simulink model "saturn_thermal5"  (R2021a)
settings: Solver=ode23t  StartTime=0.0  StopTime=t_simul  MaxStep=3600  MinStep=1  RelTol=0.1
values from neighbouring files (symbols this model uses):
  Ab = L*l    [Data_ini_thermal_analysis4.m]    (also in Data_ini_thermal_analysis5.m)
  Ant_Heater_MaxPower = 250    [Data_ini_thermal_analysis5.m]
  As = l*l    [Data_ini_thermal_analysis4.m]    (also in Data_ini_thermal_analysis5.m)
  D_st = 1224526    [Data_ini_thermal_analysis4.m]    (also in Data_ini_thermal_analysis5.m)
  ecc_sc = 0    [Data_ini_thermal_analysis4.m]    (also in Data_ini_thermal_analysis5.m)
  ecc_t = 0.0293    [Data_ini_thermal_analysis4.m]    (also in Data_ini_thermal_analysis5.m)
  Gr_al = sigma*epsilon_al*F_ds    (= 4.3092e-08)    [Data_ini_thermal_analysis4.m]    (also in Data_ini_thermal_analysis5.m)
  incl_ax_s = deg2rad(26.73)    [Data_ini_thermal_analysis4.m]    (also in Data_ini_thermal_analysis5.m)
  incl_sc = deg2rad(90+45)    [Data_ini_thermal_analysis4.m]    (also in Data_ini_thermal_analysis5.m)
  incl_t = deg2rad(0.3485)    [Data_ini_thermal_analysis4.m]    (also in Data_ini_thermal_analysis5.m)
  mean_motion_sc = 2*pi/period_sc    [Data_ini_thermal_analysis4.m]    (also in Data_ini_thermal_analysis5.m)
  mean_motion_t = (2*pi)/period_t    (= 4.56068561416e-06)    [Data_ini_thermal_analysis4.m]    (also in Data_ini_thermal_analysis5.m)
  mean_r_s = 1.427*10^9    (= 1427000000)    [Data_ini_thermal_analysis4.m]    (also in Data_ini_thermal_analysis5.m)
  mu_s = 37931187    [Data_ini_thermal_analysis4.m]    (also in Data_ini_thermal_analysis5.m)
  mu_t = 8971.15    [Data_ini_thermal_analysis4.m]    (also in Data_ini_thermal_analysis5.m)
  period_s = 29.45*365*24*3600    (= 928735200)    [Data_ini_thermal_analysis4.m]    (also in Data_ini_thermal_analysis5.m)
  period_t = 15.945421*24*3600    (= 1377684.3744)    [Data_ini_thermal_analysis4.m]    (also in Data_ini_thermal_analysis5.m)
  R_s = diam_s/2    (= 60268)    [Data_ini_thermal_analysis4.m]    (also in Data_ini_thermal_analysis5.m)
  R_t = 2576    [Data_ini_thermal_analysis4.m]    (also in Data_ini_thermal_analysis5.m)
  rho_al = 0.00277*10^6    (= 2770)    [Data_ini_thermal_analysis4.m]    (also in Data_ini_thermal_analysis5.m)
  semajax_sc = 1500+R_t    (= 4076)    [Data_ini_thermal_analysis4.m]    (also in Data_ini_thermal_analysis5.m)
  semajax_t = 1221830    [Data_ini_thermal_analysis4.m]    (also in Data_ini_thermal_analysis5.m)
  T_ds = 3    [Data_ini_thermal_analysis4.m]    (also in Data_ini_thermal_analysis5.m)
  Vol = 5    [Data_ini_thermal_analysis4.m]    (also in Data_ini_thermal_analysis5.m = 1.3)
libraries: fl_lib x273, nesl_utility x23, pid_lib x2
(part 3 of 3)

== system saturn_thermal5/Subsystem/Eclipses System1/Sun-Titan-SC/Orbit Parameter1/Inertial Orbit Direction (Theta) ==
  note: definition of orbital path:
      |
      | cos(theta(t)) position wrt X_inertial (Gamma line for example)
      |
      | sin(theta(t))*cos(i) position wrt the Y_inertial
      |
      | sin(theta(t))*sin(i) position wrt the Z-inertial
      |
      | This vector define the s/c postition around the earth
  Theta : Inport
  Constant : Constant  Value=incl_sc
  Mux : Mux  Inputs=3
  Product : Product
  Product1 : Product
  Scope : Scope
  Trigonometric Function : Trigonometry
  Trigonometric Function1 : Trigonometry  Operator=cos
  Trigonometric Function2 : Trigonometry
  Trigonometric Function3 : Trigonometry  Operator=cos
  Trigonometric Function4 : Trigonometry
  r_vn : Outport
  wires:
  Product/1 -> Mux/2
  Product1/1 -> Mux/3
  Theta/1 -> Trigonometric Function1/1, Trigonometric Function/1, Trigonometric Function2/1
  Constant/1 -> Trigonometric Function3/1, Trigonometric Function4/1
  Trigonometric Function/1 -> Product/1
  Trigonometric Function1/1 -> Mux/1
  Trigonometric Function3/1 -> Product/2
  Trigonometric Function2/1 -> Product1/1
  Trigonometric Function4/1 -> Product1/2
  Mux/1 -> Scope/1, r_vn/1

== system saturn_thermal5/Subsystem/Eclipses System1/Sun-Titan-SC/Orbit Parameter1/Inertial Orbit Radius(Theta) ==
  note: Orbital Radius magnitude computed as function of theta:
      |
      | R= a(1-ecc^2)/(1+ ecc*cos(theta(t))
  Theta : Inport
  Add : Sum
  Constant10 : Constant  Value=ecc_sc
  Constant3 : Constant  Value=semajax_sc
  Constant5 : Constant  Value=(1 - ecc_sc^2)
  Constant9 : Constant
  Divide1 : Product  Inputs=*/
  Product : Product
  Product1 : Product
  Trigonometric Function1 : Trigonometry  Operator=cos
  r_mn : Outport
  wires:
  Product1/1 -> Add/2
  Add/1 -> Divide1/2
  Divide1/1 -> r_mn/1
  Constant9/1 -> Add/1
  Trigonometric Function1/1 -> Product1/2
  Constant5/1 -> Product/2
  Product/1 -> Divide1/1
  Theta/1 -> Trigonometric Function1/1
  Constant10/1 -> Product1/1
  Constant3/1 -> Product/1

== system saturn_thermal5/Subsystem/Eclipses System1/Sun-Titan-SC/Orbit Parameter1/Subsystem ==
  r_mn : Inport
  Add : Sum  Inputs=+-
  Constant1 : Constant  Value=mu_t
  Constant2 : Constant  Value=2
  Constant4 : Constant  Value=1/semajax_sc
  Divide : Product  Inputs=**
  Divide1 : Product  Inputs=*/
  Divide2 : Product  Inputs=*/
  Scope : Scope
  Scope1 : Scope
  Square Root : Sqrt  SaturateOnIntegerOverflow=on
  wires:
  Add/1 -> Divide/2
  Constant2/1 -> Divide2/1
  Constant1/1 -> Divide/1
  Divide2/1 -> Add/1
  Constant4/1 -> Add/2
  Divide/1 -> Square Root/1
  r_mn/1 -> Divide1/2, Divide2/2
  Square Root/1 -> Divide1/1, Scope/1  "v_orb"
  Divide1/1 -> Scope1/1  "w_orb"

== system saturn_thermal5/Subsystem/Eclipses System1/Sun-Titan-SC/Orbit Parameter1/True anomaly integration ==
  Add1 : Sum
  Add2 : Sum  Inputs=+-
  Constant1 : Constant  Value=ecc_sc
  Constant7 : Constant
  Constant8 : Constant  Value=3/2
  Divide2 : Product  Inputs=*/
  Gain : Gain  Gain=ecc_sc
  Gain1 : Gain  Gain=mean_motion_sc
  Integrator : Integrator
  Math Function : Math  Operator=pow  SaturateOnIntegerOverflow=on
  Math Function1 : Math  Operator=square  SaturateOnIntegerOverflow=on
  Math Function2 : Math  Operator=square  SaturateOnIntegerOverflow=on
  Scope : Scope
  Trigonometric Function : Trigonometry  Operator=cos
  Theta : Outport
  wires:
  Gain/1 -> Add1/1
  Constant7/1 -> Add1/2, Add2/1
  Integrator/1 -> Trigonometric Function/1, Scope/1, Theta/1  "Theta"
  Divide2/1 -> Integrator/1  "Theta_dot"
  Add1/1 -> Math Function1/1
  Math Function/1 -> Divide2/2
  Trigonometric Function/1 -> Gain/1
  Gain1/1 -> Divide2/1
  Constant8/1 -> Math Function/2
  Math Function1/1 -> Gain1/1
  Constant1/1 -> Math Function2/1
  Math Function2/1 -> Add2/2
  Add2/1 -> Math Function/1
